simulink model "circuito2branch_working"  (R2018a)
settings: Solver=VariableStepAuto  StartTime=0  StopTime=102800  RelTol=1e-3
values from neighbouring files (symbols this model uses):
  A = [-1/(R1*C1),0,0;0,-1/(R2*C2),0;0,0,0]    [KF25degC_5Pulse_HPPC_Pan18650PF.m]    (also in kmfilterlcio.m)
  B = [1/C1,1/C2,-1/(Capacidad_nom*3600)]'    [KF25degC_5Pulse_HPPC_Pan18650PF.m]    (also in kmfilterlcio.m)
  C = [-1,-1,K_e]    [KF25degC_5Pulse_HPPC_Pan18650PF.m]    (also in kmfilterlcio.m)
  C1 = Tp(1)/R1    [KF25degC_5Pulse_HPPC_Pan18650PF.m]    (also in Parametros_1.mat = 7.03825015904; Parametros_2.mat = 7.45808260178)
  C2 = Tp(2)/R2    [KF25degC_5Pulse_HPPC_Pan18650PF.m]    (also in Parametros_1.mat = 556.44212235; Parametros_2.mat = 628.175708806)
  D = -R0    (= -0.02544271)    [KF25degC_5Pulse_HPPC_Pan18650PF.m]    (also in kmfilterlcio.m = -R0)
  OCV = OCV_0 + K_e*SOC    [KF25degC_5Pulse_HPPC_Pan18650PF.m]    (also in kmfilterlcio.m)
  OCV_0 = coef(2)    [KF25degC_5Pulse_HPPC_Pan18650PF.m]    (also in kmfilterlcio.m)
  R = 100    [KF25degC_5Pulse_HPPC_Pan18650PF.m]    (also in kmfilterlcio.m = 1000)
  R0 = 0.0266-0.00115729    (= 0.02544271)    [KF25degC_5Pulse_HPPC_Pan18650PF.m]    (also in Parametros_1.mat = 0.0266; Parametros_2.mat)
  R1 = Kp-R2    [KF25degC_5Pulse_HPPC_Pan18650PF.m]    (also in Parametros_1.mat = 0.0119262057484; Parametros_2.mat = 0.0130445196857)
  R2 = Kp*(Tz-Tp(2))/(Tp(1)-Tp(2))    [KF25degC_5Pulse_HPPC_Pan18650PF.m]    (also in Parametros_1.mat = 0.0135737942516; Parametros_2.mat = 0.0132554803143)
  Time = meas.Time    [KF25degC_5Pulse_HPPC_Pan18650PF.m]
  X0 = [0 0 1]    [kmfilterlcio.m]
undefined symbols (not defined in the file or in its folder): Continuous
libraries: powerlib x8, ctrlSharedLib x1
settings Model: Creator=Martin  LastModifiedBy=Martin

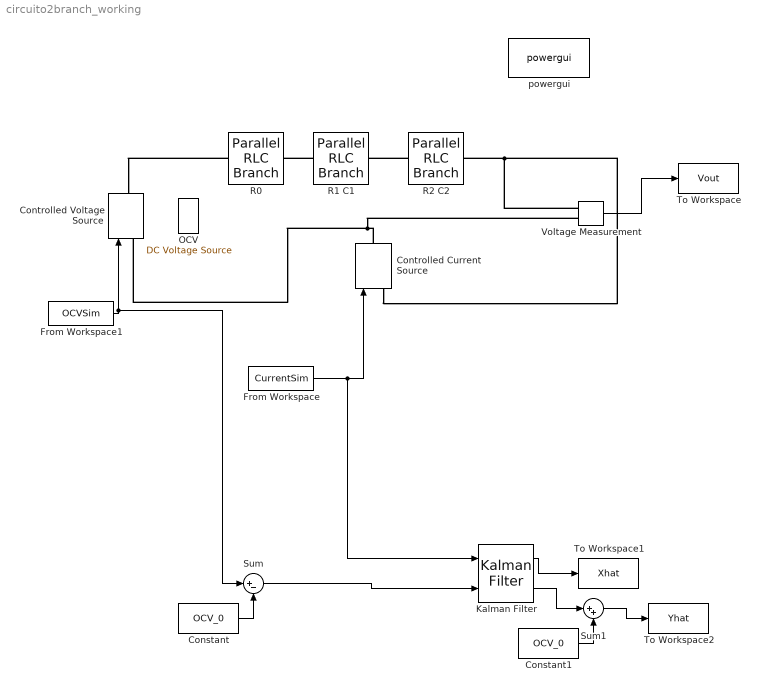
== system circuito2branch_working ==
  Constant : Constant  Value=OCV_0
  Constant1 : Constant  Value=OCV_0
  Controlled Current Source : powerlib/Electrical Sources/Controlled Current Source  Initialize=on  Source_Type=DC  Amplitude=0  Phase=0  Frequency=0  Measurements=Current
  Controlled Voltage Source : powerlib/Electrical Sources/Controlled Voltage Source  Initialize=on  Source_Type=DC  Amplitude=OCV(1)  Phase=0  Frequency=0  Measurements=None
  From Workspace : FromWorkspace  VariableName=CurrentSim  SampleTime=0
  From Workspace1 : FromWorkspace  VariableName=OCVSim  SampleTime=0
  Kalman Filter : ctrlSharedLib/Kalman Filter  TimeDomain=Continuous-Time  UseCurrentEstimator=on  ModelSource=Individual A, B, C, D matrices  ModelSourceVariable=sys  A=A  B=B  C=C  D=D  NumberOfStates=2  NumberOfInputs=2  NumberOfOutputs=2  InitialEstimateSource=Dialog  X0=X0  P0=10  UseK=off  UseGH=off  NumberOfProcessNoiseInputs=2  G=1  TimeInvariantG=on  H=0  TimeInvariantH=on  Q=Q  TimeInvariantQ=on  R=R  TimeInvariantR=on  N=0  TimeInvariantN=on  AddInputPort=on  AddEnablePort=off  OutputEstimatedY=on  OutputP=off  Ts=-1
      settings: SourceProductBaseCode=CT
  OCV : powerlib/Electrical Sources/DC Voltage Source  Amplitude=OCV  Measurements=None
  R0 : powerlib/Elements/Parallel RLC Branch  LConnTagsString=a  RConnTagsString=__new0  BranchType=R  Resistance=R0  Inductance=0  SetiL0=off  InitialCurrent=0  Capacitance=C1  Setx0=off  InitialVoltage=0  Measurements=Branch voltage
  R1 C1 : powerlib/Elements/Parallel RLC Branch  LConnTagsString=a  RConnTagsString=__new0  BranchType=RC  Resistance=R1  Inductance=0  SetiL0=off  InitialCurrent=0  Capacitance=C1  Setx0=on  InitialVoltage=0  Measurements=Branch voltage
  R2 C2 : powerlib/Elements/Parallel RLC Branch  LConnTagsString=a  RConnTagsString=__new0  BranchType=RC  Resistance=R2  Inductance=0  SetiL0=off  InitialCurrent=0  Capacitance=C2  Setx0=on  InitialVoltage=0  Measurements=Branch voltage
  Sum : Sum  Inputs=|+-
  Sum1 : Sum  Inputs=|++
  To Workspace : ToWorkspace  VariableName=Vout  SaveFormat=Timeseries  SampleTime=-1
  To Workspace1 : ToWorkspace  VariableName=Xhat  SaveFormat=Timeseries  SampleTime=-1
  To Workspace2 : ToWorkspace  VariableName=Yhat  SaveFormat=Timeseries  SampleTime=-1
  Voltage Measurement : powerlib/Measurements/Voltage Measurement  PhasorSimulation=off  OutputType=Complex  PSBequivalent=0
  powergui : powerlib/powergui  Priority=1  SimulationMode=Continuous  SampleTime=50e-6  frequency=60  Iterations=50  frequencyindice=0  Pbase=100e6  ErrMax=1e-4  UnitsV=kV  UnitsW=MW  buscounter=0  FunctionMessages=off  echomessages=off  EnableUseOfTLC=off  CurrentSourceSwitches=off  DisableSnubberDevices=off  DisableRonSwitches=off  DisableVfSwitches=off  DisplayEquations=off  SolverType=Tustin/Backward Euler (TBE)  Interpol=off  ExternalGateDelay=off  methode=off  Ts=100  x0status=blocks  SPID=on  SwTol=0  HookPort=off  RestoreLinks=warning  ResistiveCurrentMeasurement=off  Frange=[0:2:500]  Ylog=off  Xlog=on  ShowGrid=off  save=off  variable=ZData  structure=0  ZoomFFT=off  StartTime=0.0  cycles=1  DisplayStyle=1  fundamental=60  FreqAxis=off  MaxFrequency=1000  frequencyindicesteady=1  RmsSteady=1  display=off
  wires:
  Voltage Measurement/1 -> To Workspace/1
  From Workspace1/1 -> Sum/1, Controlled Voltage Source/1
  From Workspace/1 -> Kalman Filter/1, Controlled Current Source/1
  Kalman Filter/1 -> To Workspace1/1
  Sum/1 -> Kalman Filter/2
  Constant/1 -> Sum/2
  Constant1/1 -> Sum1/2
  Sum1/1 -> To Workspace2/1
  Kalman Filter/2 -> Sum1/1
  connections:
  R2 C2/LConn1 -- R1 C1/RConn1
  Controlled Current Source/RConn1 -- Controlled Voltage Source/LConn1 -- Voltage Measurement/LConn2
  R1 C1/LConn1 -- R0/RConn1
  Controlled Current Source/LConn1 -- Voltage Measurement/LConn1 -- R2 C2/RConn1
  R0/LConn1 -- Controlled Voltage Source/RConn1
